simulink model "DistanceStepResponse"  (R2021a)
settings: Solver=VariableStepAuto  StartTime=0.0  StopTime=20.0  RelTol=1e-3
values from neighbouring files (symbols this model uses):
  K = 0.057    [ForwardVelStepEx.m]
  sigma = 5    [ForwardVelStepEx.m]
settings Model: Creator=nolanegging  LastModifiedBy=LWag
settings SolverCC: AlgebraicLoopSolver=TrustRegion
settings DebuggingCC: SFMachineParentedDataDiag=warning

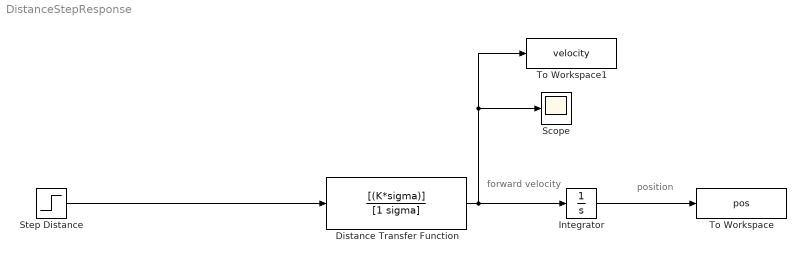
== system DistanceStepResponse ==
  note: position
  note: forward velocity
  Distance Transfer Function : TransferFcn  Numerator=[(K*sigma)]  Denominator=[1 sigma]
  Integrator : Integrator
  Scope : Scope
  Step Distance : Step  After=5  SampleTime=0
  To Workspace : ToWorkspace  VariableName=pos  SaveFormat=Timeseries  SampleTime=-1
  To Workspace1 : ToWorkspace  VariableName=velocity  SaveFormat=Timeseries  SampleTime=-1
  wires:
  Distance Transfer Function/1 -> Integrator/1, Scope/1, To Workspace1/1
  Integrator/1 -> To Workspace/1
  Step Distance/1 -> Distance Transfer Function/1
